simulink model "InvertedPendulumNM"  (R2017a)
settings: Solver=VariableStepAuto  StartTime=0.0  StopTime=tf  RelTol=1e-3
values from neighbouring files (symbols this model uses):
  b = 0.1    [Inverted_pendulum.m]    (also in euler.m; inv_pend.m)
  g = 9.8    [Inverted_pendulum.m]    (also in euler.m = 9.807; inv_pend.m)
  I = 0.006    [Inverted_pendulum.m]    (also in euler.m; inv_pend.m)
  L = 0.3    [Inverted_pendulum.m]    (also in euler.m)
  M = 0.5    [Inverted_pendulum.m]    (also in euler.m; inv_pend.m)
  m = 0.2    [Inverted_pendulum.m]    (also in euler.m; inv_pend.m)
settings Model: Creator=aposad31  LastModifiedBy=santiago

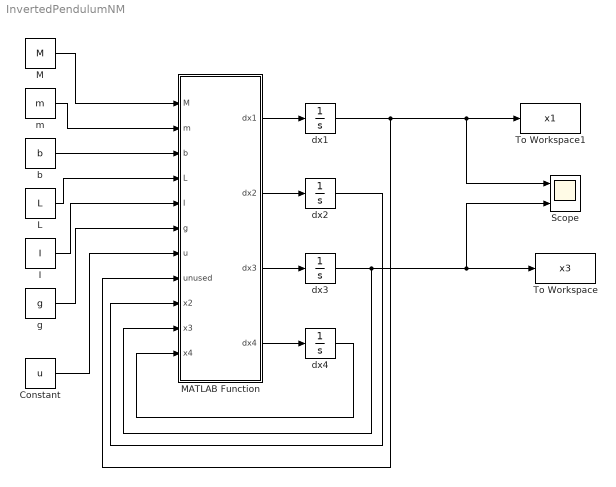
== system InvertedPendulumNM ==
  Constant : Constant  Value=u
  I : Constant  Value=I
  L : Constant  Value=L
  M : Constant  Value=M
  MATLAB Function : MATLAB Function  TreatAsAtomicUnit=on
  Scope : Scope  NumInputPorts=2
  To Workspace : ToWorkspace  VariableName=x3  SaveFormat=Timeseries  SampleTime=-1
  To Workspace1 : ToWorkspace  VariableName=x1  SaveFormat=Timeseries  SampleTime=-1
  b : Constant  Value=b
  dx{1..4} (4 alike) : Integrator
  g : Constant  Value=g
  m : Constant  Value=m
  wires:
  dx3/1 -> To Workspace/1, Scope/2, MATLAB Function/10(x3)
  dx1/1 -> MATLAB Function/8(unused), To Workspace1/1, Scope/1
  I/1 -> MATLAB Function/5(I)
  L/1 -> MATLAB Function/4(L)
  g/1 -> MATLAB Function/6(g)
  dx2/1 -> MATLAB Function/9(x2)
  MATLAB Function/4(dx4) -> dx4/1
  b/1 -> MATLAB Function/3(b)
  M/1 -> MATLAB Function/1(M)
  MATLAB Function/3(dx3) -> dx3/1
  dx4/1 -> MATLAB Function/11(x4)
  MATLAB Function/1(dx1) -> dx1/1
  m/1 -> MATLAB Function/2(m)
  MATLAB Function/2(dx2) -> dx2/1
  Constant/1 -> MATLAB Function/7(u)

== matlab function InvertedPendulumNM/MATLAB Function ==
  data: M input; m input; b input; L input; I input; g input; u input; dx1 output; unused input; x2 input; x3 input; x4 input; dx2 output; dx3 output; dx4 output
function [dx1, dx2, dx3, dx4] = fcn(M, m, b, L, I, g, u, ~, x2, x3, x4)
    denominator = (M+m).*(I+m.*L.^2)-m.^2.*L.^2.*cos(x3).^2;
    dx1 = x2;
    dx2 = ((I+m.*L.^2).*(u-b.*x2+m.*L.*x4.^2.*sin(x3))+m.^2.*L.^2.*g.*sin(x3).*cos(x3))./denominator;
    dx3 = x4;
    dx4 = (-m.*L.*u.*cos(x3)+m.*L.*b.*x2.*cos(x3)-m.^2.*L.^2.*x4.^2.*sin(x3).*cos(x3)-(M+m).*m*g.*L.*sin(x3))./denominator;
end
